simulink model "ECBtn_VD"  (R2016b)
settings: configuration reference "CodeGenConfigSet" (kept outside this file)
settings Model: Creator=xinchangran  LastModifiedBy=xinchangran
settings ConfigSetRef: SourceLocation=Base Workspace

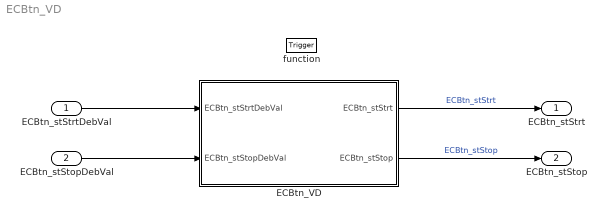
== system ECBtn_VD ==
  ECBtn_stStrtDebVal : Inport  Description=start signal  OutMin=0  OutMax=1  OutDataTypeStr=boolean
  ECBtn_stStopDebVal : Inport  Description=stop signal  Port=2  OutMin=0  OutMax=1  OutDataTypeStr=boolean
  function : TriggerPort  TriggerType=function-call  VariantControl=Variant
  ECBtn_VD : Subsystem
  ECBtn_stStrt : Outport  Description=start state Virtual Device out  OutMin=0  OutMax=1  OutDataTypeStr=boolean
  ECBtn_stStop : Outport  Description=stop state Virtual Device out  Port=2  OutMin=0  OutMax=1  OutDataTypeStr=boolean
  wires:
  ECBtn_stStrtDebVal/1 -> ECBtn_VD/1(ECBtn_stStrtDebVal)
  ECBtn_stStopDebVal/1 -> ECBtn_VD/2(ECBtn_stStopDebVal)
  ECBtn_VD/1(ECBtn_stStrt) -> ECBtn_stStrt/1  "ECBtn_stStrt"
  ECBtn_VD/2(ECBtn_stStop) -> ECBtn_stStop/1  "ECBtn_stStop"

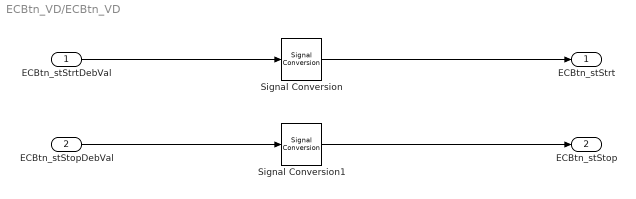
== system ECBtn_VD/ECBtn_VD ==
  ECBtn_stStrtDebVal : Inport  Description=start signal  OutMin=0  OutMax=1  OutDataTypeStr=boolean
  ECBtn_stStopDebVal : Inport  Description=stop signal  Port=2  OutMin=0  OutMax=1  OutDataTypeStr=boolean
  Signal Conversion : SignalConversion  OverrideOpt=off
  Signal Conversion1 : SignalConversion  OverrideOpt=off
  ECBtn_stStrt : Outport  Description=start state Virtual Device out  OutMin=0  OutMax=1  OutDataTypeStr=boolean
  ECBtn_stStop : Outport  Description=stop state Virtual Device out  Port=2  OutMin=0  OutMax=1  OutDataTypeStr=boolean
  wires:
  ECBtn_stStrtDebVal/1 -> Signal Conversion/1
  ECBtn_stStopDebVal/1 -> Signal Conversion1/1
  Signal Conversion1/1 -> ECBtn_stStop/1
  Signal Conversion/1 -> ECBtn_stStrt/1
